simulink model "LLC_Controller"  (R2022b)
settings: Solver=FixedStepDiscrete  StartTime=0.0  StopTime=Inf  FixedStep=(20e-6)  RelTol=1e-3  EnableMultiTasking=on
undefined symbols (not defined in the file): GPTRIP1SEL, GPTRIP2SEL, SCI_A_Transmit, SCI_A_Transmit_Current_Suffix, SCI_A_Transmit_Duty_Suffix, SCI_A_Transmit_Freq_Suffix, SCI_A_Transmit_NewVRegPoint_Suffix, SCI_A_Transmit_OCPFlag_Suffix, SCI_A_Transmit_OVPFlag_Suffix, SCI_A_Transmit_PFC_Suffix, SCI_A_Transmit_SS_Suffix, SCI_A_Transmit_TBPHS_Suffix, SCI_A_Transmit_VADC_Suffix, SCI_A_Transmit_VAvg_Suffix, SCI_A_Transmit_VBAT_Suffix, SCI_A_Transmit_VBATRef_Suffix, SCI_A_Transmit_Vo_Suffix, TZ1, TZ2
libraries: c280xlib x16, c28003xlib x13, c2802xlib x8, simulink x7, c2837xDlib x3, c2000lib x1
(part 1 of 2)
settings Model: ExtModeTrigDuration=8  Creator=sgcesuser1  LastModifiedBy=sgcesuser1
settings SolverCC: AutoInsertRateTranBlk=on
settings DataIOCC: LimitDataPoints=on  SaveOutput=off  SaveTime=off  ReturnWorkspaceOutputs=off
settings OptimizationCC: DefaultUnderspecifiedDataType=single  EnhancedBackFolding=on  PassReuseOutputArgsAs=Individual arguments  MaxStackSize=1024  OptimizeBlockOrder=speed  DifferentSizesBufferReuse=on  OptimizationCustomize=off  DenormalBehavior=FlushToZero  EfficientTunableParamExpr=on
settings DebuggingCC: SolverPrmCheckMsg=warning  MultiTaskDSMMsg=none  MultiTaskCondExecSysMsg=none  ParameterTunabilityLossMsg=error  UnconnectedInputMsg=warning  UnconnectedOutputMsg=warning  UnconnectedLineMsg=warning  StateNameClashWarn=warning  SFUnexpectedBacktrackingDiag=warning  SFNoUnconditionalDefaultTransitionDiag=warning
settings HardwareCC: ProdBitPerChar=16  ProdBitPerInt=16  ProdBitPerPointer=32  ProdBitPerSizeT=32  ProdBitPerPtrDiffT=32  ProdLargestAtomicInteger=Integer  ProdLargestAtomicFloat=None  ProdWordSize=16  ProdLongLongMode=on  ProdHWDeviceType=Texas Instruments->C2000
settings ModelReferenceCC: EnableRefExpFcnMdlSchedulingChecks=on  PropagateSignalLabelsOutOfModel=off
settings SFSimCC: MATLABDynamicMemAlloc=off
settings RTWCC: Description=Embedded Coder  SystemTargetFile=ert.tlc  HardwareBoard=TI F28003x  TLCOptions=-aInlineSetEventsForThisBaseRateFcn=TLC_FALSE -aSuppressMultiTaskScheduler=TLC_FALSE -aRateBasedStepFcn=1  TemplateMakefile=ert_default_tmf  GenerateReport=on  Toolchain=Texas Instruments Code Composer Studio (C2000)  LaunchReport=on
settings CodeAppCC: IgnoreCustomStorageClasses=off  StateflowObjectComments=on
settings ERTTargetCC: CodeReplacementLibrary=TI C28x  ExtModeTransport=4  ExtModeStaticAlloc=on  ExtModeMexFile=ext_xcp  ExtModeIntrfLevel=Level2 - Open  ConvertIfToSwitch=off  SuppressUnreachableDefaultCases=off

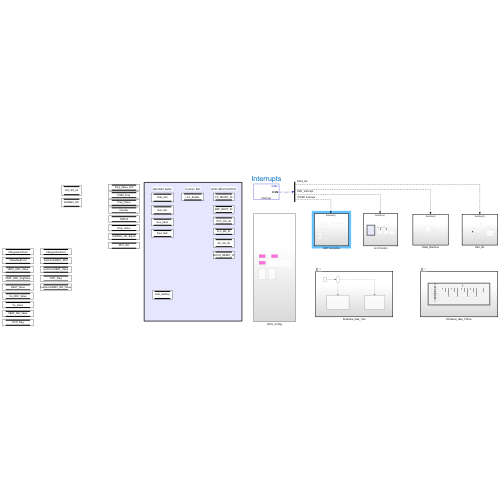
[thumbnail: Simulink's stored preview of the top-level diagram]
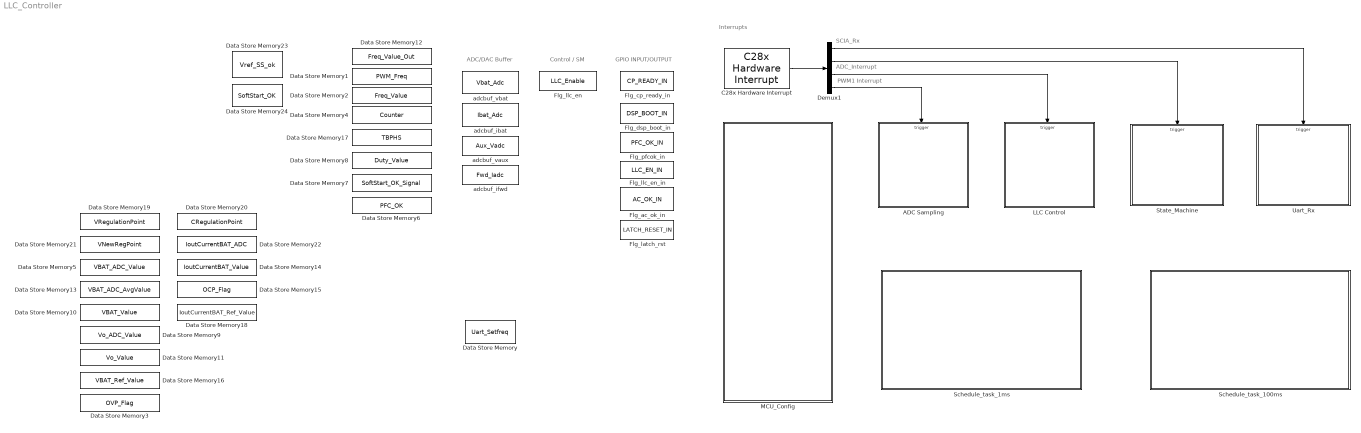
== system LLC_Controller ==
  note: ADC_Interrupt
  note: PWM1 Interrupt
  note: Interrupts
  note: GPIO INPUT/OUTPUT
  note: ADC/DAC Buffer
  note: Control / SM
  note: SCIA_Rx
  ADC Sampling : Subsystem  TreatAsAtomicUnit=on
  C28x Hardware Interrupt : c2000lib/Scheduling/C28x Hardware Interrupt  irqnumbers=[9 3 1 3]  pienumbers=[1 8 3 1]  irqpriorities=[33 32 30 31]  irqpreempts=[1 1 0 0]  showinput=off  dspchiptype=C280X
  Data Store Memory : DataStoreMemory  DataStoreName=Uart_Setfreq  WriteAfterWriteMsg=warning  InitialValue=100  ShowAdditionalParam=off  OutDataTypeStr=single
  Data Store Memory1 : DataStoreMemory  DataStoreName=PWM_Freq  WriteAfterWriteMsg=warning  ShowAdditionalParam=off  OutDataTypeStr=double
  Data Store Memory10 : DataStoreMemory  DataStoreName=VBAT_Value  WriteAfterWriteMsg=warning  ShowAdditionalParam=off  OutDataTypeStr=double
  Data Store Memory11 : DataStoreMemory  DataStoreName=Vo_Value  WriteAfterWriteMsg=warning  InitialValue=153  ShowAdditionalParam=off
  Data Store Memory12 : DataStoreMemory  DataStoreName=Freq_Value_Out  WriteAfterWriteMsg=warning  InitialValue=153  ShowAdditionalParam=off  OutDataTypeStr=double
  Data Store Memory13 : DataStoreMemory  DataStoreName=VBAT_ADC_AvgValue  WriteAfterWriteMsg=warning  ShowAdditionalParam=off
  Data Store Memory14 : DataStoreMemory  DataStoreName=IoutCurrentBAT_Value  WriteAfterWriteMsg=warning  ShowAdditionalParam=off  OutDataTypeStr=double
  Data Store Memory15 : DataStoreMemory  DataStoreName=OCP_Flag  WriteAfterWriteMsg=warning  InitialValue=1  ShowAdditionalParam=off
  Data Store Memory16 : DataStoreMemory  DataStoreName=VBAT_Ref_Value  WriteAfterWriteMsg=warning  ShowAdditionalParam=off  OutDataTypeStr=double
  Data Store Memory17 : DataStoreMemory  DataStoreName=TBPHS  WriteAfterWriteMsg=warning  ShowAdditionalParam=off  OutDataTypeStr=double
  Data Store Memory18 : DataStoreMemory  DataStoreName=IoutCurrentBAT_Ref_Value  WriteAfterWriteMsg=warning  ShowAdditionalParam=off  OutDataTypeStr=double
  Data Store Memory19 : DataStoreMemory  DataStoreName=VRegulationPoint  WriteAfterWriteMsg=warning  ShowAdditionalParam=off  OutDataTypeStr=double
  Data Store Memory2 : DataStoreMemory  DataStoreName=Freq_Value  WriteAfterWriteMsg=warning  InitialValue=153  ShowAdditionalParam=off  OutDataTypeStr=double
  Data Store Memory20 : DataStoreMemory  DataStoreName=CRegulationPoint  WriteAfterWriteMsg=warning  ShowAdditionalParam=off  OutDataTypeStr=double
  Data Store Memory21 : DataStoreMemory  DataStoreName=VNewRegPoint  WriteAfterWriteMsg=warning  ShowAdditionalParam=off  OutDataTypeStr=double
  Data Store Memory22 : DataStoreMemory  DataStoreName=IoutCurrentBAT_ADC  WriteAfterWriteMsg=warning  ShowAdditionalParam=off  OutDataTypeStr=double
  Data Store Memory23 : DataStoreMemory  DataStoreName=Vref_SS_ok  WriteAfterWriteMsg=warning  ShowAdditionalParam=off
  Data Store Memory24 : DataStoreMemory  DataStoreName=SoftStart_OK  WriteAfterWriteMsg=warning  ShowAdditionalParam=off
  Data Store Memory3 : DataStoreMemory  DataStoreName=OVP_Flag  WriteAfterWriteMsg=warning  InitialValue=1  ShowAdditionalParam=off
  Data Store Memory4 : DataStoreMemory  DataStoreName=Counter  WriteAfterWriteMsg=warning  InitialValue=153  ShowAdditionalParam=off
  Data Store Memory5 : DataStoreMemory  DataStoreName=VBAT_ADC_Value  WriteAfterWriteMsg=warning  InitialValue=153  ShowAdditionalParam=off  OutDataTypeStr=double
  Data Store Memory6 : DataStoreMemory  DataStoreName=PFC_OK  WriteAfterWriteMsg=warning  ShowAdditionalParam=off
  Data Store Memory7 : DataStoreMemory  DataStoreName=SoftStart_OK_Signal  WriteAfterWriteMsg=warning  ShowAdditionalParam=off
  Data Store Memory8 : DataStoreMemory  DataStoreName=Duty_Value  WriteAfterWriteMsg=warning  InitialValue=1  ShowAdditionalParam=off  OutDataTypeStr=double
  Data Store Memory9 : DataStoreMemory  DataStoreName=Vo_ADC_Value  WriteAfterWriteMsg=warning  InitialValue=153  ShowAdditionalParam=off
  Demux1 : Demux
  Flg_ac_ok_in : DataStoreMemory  DataStoreName=AC_OK_IN  WriteAfterWriteMsg=warning  ShowAdditionalParam=off
  Flg_cp_ready_in : DataStoreMemory  DataStoreName=CP_READY_IN  WriteAfterWriteMsg=warning  ShowAdditionalParam=off
  Flg_dsp_boot_in : DataStoreMemory  DataStoreName=DSP_BOOT_IN  WriteAfterWriteMsg=warning  ShowAdditionalParam=off
  Flg_latch_rst : DataStoreMemory  DataStoreName=LATCH_RESET_IN  WriteAfterWriteMsg=warning  ShowAdditionalParam=off
  Flg_llc_en : DataStoreMemory  DataStoreName=LLC_Enable  WriteAfterWriteMsg=warning  ShowAdditionalParam=off  OutDataTypeStr=boolean
  Flg_llc_en_in : DataStoreMemory  DataStoreName=LLC_EN_IN  WriteAfterWriteMsg=warning  ShowAdditionalParam=off
  Flg_pfcok_in : DataStoreMemory  DataStoreName=PFC_OK_IN  WriteAfterWriteMsg=warning  ShowAdditionalParam=off
  LLC Control : Subsystem  TreatAsAtomicUnit=on
  MCU_Config : Subsystem
  Schedule_task_100ms : Subsystem  TreatAsAtomicUnit=on  ScheduleAs=Periodic partition  PartitionName=Schedule_task_100ms  SystemSampleTime=1
  Schedule_task_1ms : Subsystem  TreatAsAtomicUnit=on  ScheduleAs=Periodic partition  PartitionName=Schedule_task_1ms  SystemSampleTime=0.001
  State_Machine : Subsystem  TreatAsAtomicUnit=on
  Uart_Rx : Subsystem  TreatAsAtomicUnit=on
  adcbuf_ibat : DataStoreMemory  DataStoreName=Ibat_Adc  WriteAfterWriteMsg=warning  ShowAdditionalParam=off  OutDataTypeStr=uint16
  adcbuf_ifwd : DataStoreMemory  DataStoreName=Fwd_Iadc  WriteAfterWriteMsg=warning  ShowAdditionalParam=off  OutDataTypeStr=uint16
  adcbuf_vaux : DataStoreMemory  DataStoreName=Aux_Vadc  WriteAfterWriteMsg=warning  ShowAdditionalParam=off  OutDataTypeStr=uint16
  adcbuf_vbat : DataStoreMemory  DataStoreName=Vbat_Adc  WriteAfterWriteMsg=warning  ShowAdditionalParam=off  OutDataTypeStr=uint16
  wires:
  C28x Hardware Interrupt/1 -> Demux1/1
  Demux1/3 -> LLC Control/Trigger
  Demux1/4 -> ADC Sampling/Trigger
  Demux1/2 -> State_Machine/Trigger
  Demux1/1 -> Uart_Rx/Trigger

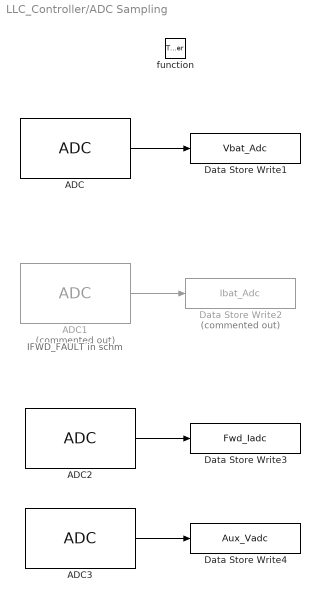
== system LLC_Controller/ADC Sampling ==
  note: IFWD_FAULT in schm
  function : TriggerPort  TriggerType=function-call  VariantControl=(inherit)
  ADC : c2802xlib/ADC  blkParamProc=C2000_Type5  ADCModule=C  samplingMode=Single sample mode  ADCResolution=12-bit (Single-ended input)  useSOC1=SOC0  useSOC2=SOC0_SOC1  SOCAcquisitionWindow=8  SOCTriggerSource=Software  SOCInterruptTrigger=No ADCINT  Ts=-1  dType=uint16  postInterrupt=on  interruptSel=ADCINT1  ADCINTContinuous=on  endma=off  chdma=1  conv1=ADCINA0  conv2=ADCINA0 and ADCINB0  conv1_Type4=ADCIN5  conv2_Type4=ADCIN0 and ADCIN1
  ADC1 : c2802xlib/ADC  Commented=on  blkParamProc=C2000_Type5  ADCModule=A  samplingMode=Single sample mode  ADCResolution=12-bit (Single-ended input)  useSOC1=SOC2  useSOC2=SOC0_SOC1  SOCAcquisitionWindow=8  SOCTriggerSource=Software  SOCInterruptTrigger=No ADCINT  Ts=-1  dType=uint16  postInterrupt=off  interruptSel=ADCINT1  ADCINTContinuous=off  endma=off  chdma=1  conv1=ADCINA0  conv2=ADCINA0 and ADCINB0  conv1_Type4=ADCIN9  conv2_Type4=ADCIN0 and ADCIN1
  ADC2 : c2802xlib/ADC  blkParamProc=C2000_Type5  ADCModule=B  samplingMode=Single sample mode  ADCResolution=12-bit (Single-ended input)  useSOC1=SOC0  useSOC2=SOC0_SOC1  SOCAcquisitionWindow=8  SOCTriggerSource=Software  SOCInterruptTrigger=No ADCINT  Ts=-1  dType=uint16  postInterrupt=off  interruptSel=ADCINT1  ADCINTContinuous=off  endma=off  chdma=1  conv1=ADCINA0  conv2=ADCINA0 and ADCINB0  conv1_Type4=ADCIN11  conv2_Type4=ADCIN0 and ADCIN1
  ADC3 : c2802xlib/ADC  blkParamProc=C2000_Type5  ADCModule=C  samplingMode=Single sample mode  ADCResolution=12-bit (Single-ended input)  useSOC1=SOC2  useSOC2=SOC0_SOC1  SOCAcquisitionWindow=8  SOCTriggerSource=Software  SOCInterruptTrigger=No ADCINT  Ts=-1  dType=uint16  postInterrupt=off  interruptSel=ADCINT1  ADCINTContinuous=off  endma=off  chdma=1  conv1=ADCINA0  conv2=ADCINA0 and ADCINB0  conv1_Type4=ADCIN1  conv2_Type4=ADCIN0 and ADCIN1
  Data Store Write1 : DataStoreWrite  DataStoreName=Vbat_Adc  IndexOptions=Index vector (dialog)  Indices=1  OutputSizes=1
  Data Store Write2 : DataStoreWrite  Commented=on  DataStoreName=Ibat_Adc  IndexOptions=Index vector (dialog)  Indices=1  OutputSizes=1
  Data Store Write3 : DataStoreWrite  DataStoreName=Fwd_Iadc  IndexOptions=Index vector (dialog)  Indices=1  OutputSizes=1
  Data Store Write4 : DataStoreWrite  DataStoreName=Aux_Vadc  IndexOptions=Index vector (dialog)  Indices=1  OutputSizes=1
  wires:
  ADC/1 -> Data Store Write1/1
  ADC1/1 -> Data Store Write2/1
  ADC2/1 -> Data Store Write3/1
  ADC3/1 -> Data Store Write4/1

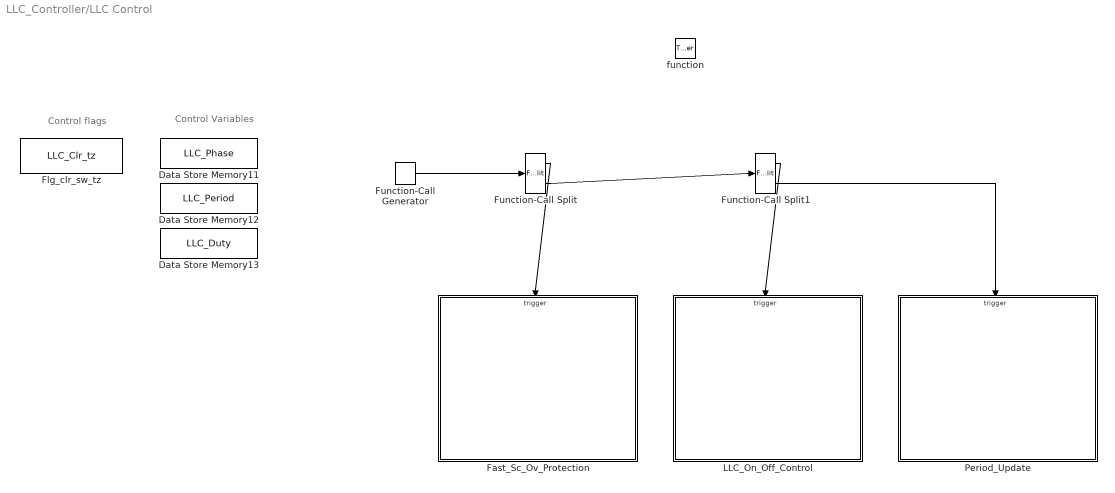
== system LLC_Controller/LLC Control ==
  note: Control flags
  note: Control Variables
  function : TriggerPort  TriggerType=function-call  VariantControl=(inherit)
  Data Store Memory11 : DataStoreMemory  DataStoreName=LLC_Phase  WriteAfterWriteMsg=warning  InitialValue=300  ShowAdditionalParam=off  OutDataTypeStr=single
  Data Store Memory12 : DataStoreMemory  DataStoreName=LLC_Period  WriteAfterWriteMsg=warning  InitialValue=(120e6)/(300e3)  ShowAdditionalParam=off  OutDataTypeStr=single
  Data Store Memory13 : DataStoreMemory  DataStoreName=LLC_Duty  WriteAfterWriteMsg=warning  InitialValue=(100/50)  ShowAdditionalParam=off  OutDataTypeStr=single
  Fast_Sc_Ov_Protection : Subsystem  TreatAsAtomicUnit=on
  Flg_clr_sw_tz : DataStoreMemory  DataStoreName=LLC_Clr_tz  WriteAfterWriteMsg=warning  ShowAdditionalParam=off  OutDataTypeStr=boolean
  Function-Call Generator : simulink/Ports & Subsystems/Function-Call Generator  sample_time=-1  numberOfIterations=1  DisallowWideOutput=off
  Function-Call Split : FunctionCallSplit  NumOutputPorts=2
  Function-Call Split1 : FunctionCallSplit  NumOutputPorts=2
  LLC_On_Off_Control : Subsystem  TreatAsAtomicUnit=on
  Period_Update : Subsystem  TreatAsAtomicUnit=on
  wires:
  Function-Call Generator/1 -> Function-Call Split/1
  Function-Call Split/1 -> Fast_Sc_Ov_Protection/Trigger
  Function-Call Split1/1 -> LLC_On_Off_Control/Trigger
  Function-Call Split/2 -> Function-Call Split1/1
  Function-Call Split1/2 -> Period_Update/Trigger

== system LLC_Controller/MCU_Config ==
  note: EALLOW;
      | EPwm5Regs.EPWMSYNCOUTEN.all = 0x02;  //PWM5 SYNCOUT signal at TBCTR = 0
      | EPwm7Regs.EPWMSYNCINSEL.all = 0x05;    //PWM7 SYNCIN to PWM5
      | EPwm5Regs.TZSEL.bit.OSHT1 = 1;
      | EPwm7Regs.TZSEL.bit.OSHT1 = 1;
      | EPwm5Regs.TZFRC.bit.OST = 1;
      | EPwm7Regs.TZFRC.bit.OST = 1;
      | EDIS;
  ADC_TriggerSource : c2802xlib/ePWM  PwmType=C2000_Type4_F28002x  useModule=ePWM1  ePWMxLINKTBPRD=Not Linked  periodUnits=Seconds  timerSource=Specify via dialog  timerPeriod_clk=(120e6/50e3)  timerPeriod_sec=50e-6  tbshadow=Counter equals to zero  countingMode=Up  phaseActiveEnable=Disable  phaseDirection=Count down after sync  phaseActive=0  synchronizationEnable=off  dcaevt1Sync=off  dcbevt1Sync=off  synchronizationOption=Counter equals to zero (CTR=Zero)  dcbevt1SyncOut=off  dcaevt1SyncOut=off  cmpdSyncOut=off  cmpcSyncOut=off  cmpbSyncOut=off  zeroSyncOut=on  swfSyncOut=off  perSynchronizationOption=Counter equals to period (CTR=PRD)  clockPrescale=1  HSclockPrescale=1  enswap=off  ePWMxAStatus=off  ePWMxAactionLogic1=Set  ePWMxAactionLogic2=Do nothing  ePWMxAactionLogic3=Clear  ePWMxAactionLogic4=Do nothing  ePWMxAactionLogic5=Do nothing  ePWMxAactionLogic6=Do nothing  ePWMxACSFenable=off  ePWMxACSFvalue=Forcing disable  ePWMxASFreload=Zero  ePWMxBStatus=off  ePWMxBactionLogic1=Clear  ePWMxBactionLogic2=Do nothing  ePWMxBactionLogic3=Set  ePWMxBactionLogic4=Do nothing  ePWMxBactionLogic5=Do nothing  ePWMxBactionLogic6=Set  ePWMxBCSFenable=off  ePWMxBCSFvalue=Forcing disable  ePWMxBSFreload=Zero  ePWNxBOutWay=off  ePWMxLINKCMPA=Not Linked  CMPAUnits=Clock cycles  CMPASource=Specify via dialog  CMPAValue_per=50  CMPAValue_clk=50  enCMPAshadow=Counter equals to zero (CTR=Zero)  ePWMxLINKCMPB=Not Linked  CMPBUnits=Clock cycles  CMPBSource=Specify via dialog  CMPBValue_per=50  CMPBValue_clk=1000  enCMPBshadow=Counter equals to zero (CTR=Zero)  ePWMxLINKCMPC=Not Linked  CMPCUnits=Clock cycles  CMPCSource=Specify via dialog  CMPCValue_per=50  CMPCValue_clk=32000  enCMPCshadow=Counter equals to zero (CTR=Zero)  ePWMxLINKCMPD=Not Linked  CMPDUnits=Percentages  CMPDSource=Specify via dialog  CMPDValue_per=50  CMPDValue_clk=32000  enCMPDshadow=Counter equals to zero (CTR=Zero)  enableDBePWMxA=off  enableDBePWMxB=off  enhalfcycle=off  DBpolarity=Active high complementary (AHC)  DBedgeDelay=Positive  DBSource_ePWMxA=ePWMxA  DBSource_ePWMxB=ePWMxA  DBPeriodUnits=Seconds  DBperiodSource=Specify via dialog  REDperiod=0  FEDperiod=0  REDperiod_sec=250e-9  FEDperiod_sec=250e-9  LoadModeDBRED=Counter equals to zero (CTR=ZERO)  LoadModeDBFED=Counter equals to zero (CTR=ZERO)  adcstartModuleA=off  adcrequestEventA=First event  adcstartEventA=Counter equals to zero (CTR=Zero)  adcstartEventA_type2=Counter equals to zero (CTR=Zero)  adcstartModuleB=off  adcrequestEventB=First event  adcstartEventB=Counter equals to zero (CTR=Zero)  adcstartEventB_type2=Counter equals to zero (CTR=Zero)  intEn=on  intPrd=First event  intSel=Counter equals to zero (CTR=Zero)  intSel_type2=Counter equals to zero (CTR=Zero)  hrpe=off  enHRPWM=off  HRPWM_LoadMode=Counter equals to zero (CTR=ZERO)  HRPWM_CTLMode=Duty or Period control mode  HRPWM_EDGMode=Both edge  hrpeb=off  enHRPWMB=off  HRPWM_LoadModeB=Counter equals to zero (CTR=ZERO)  HRPWM_CTLModeB=Duty or Period control mode  HRPWM_EDGModeB=Both edge  enHRDBRED=off  enHRDBFED=off  enSFO=on  enautoconv=on  chopperEnable=off  chopperFrequency=1  chopperFirstwidth=1  chopperDuty=12.5%  tripZonesource=Specify via dialog  tzselOSHT1=off  tzselOSHT2=off  tzselOSHT3=off  tzselOSHDCAEV1=off  tzselOSHDCBEV1=off  tzselCBC1=off  tzselCBC2=off  tzselCBC3=off  tzselCBCDCAEV2=off  tzselCBCDCBEV2=off  tzselOSHT4=off  tzselOSHT5=off  tzselOSHT6=off  tzselCBC4=off  tzselCBC5=off  tzselCBC6=off  enTzOstIntr=off  enTzCbcIntr=off  enTzDCAEVT1Intr=off  enTzDCAEVT2Intr=off  enTzDCBEVT1Intr=off  enTzDCBEVT2Intr=off  ePWMxAforced=No action  ePWMxBforced=No action  DCAEVT1forced=No action  DCBEVT1forced=No action  DCAEVT2forced=No action  DCBEVT2forced=No action  dcah=Trip Zone 1 input (TZ1)  dcal=Trip Zone 1 input (TZ1)  dcbh=Trip Zone 1 input (TZ1)  dcbl=Trip Zone 1 input (TZ1)  dcah_type2=GPTRIP1SEL/(TZ1)  dcal_type2=GPTRIP2SEL/(TZ2)  dcbh_type2=GPTRIP1SEL/(TZ1)  dcbl_type2=GPTRIP2SEL/(TZ2)  gendcaevt1=Event disabled  gendcaevt2=Event disabled  gendcbevt1=Event disabled  gendcbevt2=Event disabled  dcaevt1src=DCAEVT1 with sync  dcaevt2src=DCAEVT2 with sync  dcbevt1src=DCBEVT1 with sync  dcbevt2src=DCBEVT2 with sync  pulsesel=Counter equals to zero (CTR=Zero)  blankinv=off  blankoffset=0  blankwidth=0  evsrcsel=Filtered version of DCAEVT1 (DCAEVT1FILT)  encape=off
  CMPSS/ANALOG Initialize : Subsystem  mask(System Initialize){ShowInLibBrowser=0}
      mask prompts: ShowInLibBrowser "Simulink:masks:CustCodeMaskParam1_MP"
      settings: CopyFcn=cccopyfcn(gcb)  OpenFcn=ccopenfcn('System Initialize Function')
      mask Help: eval('feval(''rtwprivate'',''rtwhelpview'',''rtw_sys_initialize_block'')');
      mask Display: disp('System\nInitialize');
  PWM Initialize : Subsystem  mask(System Initialize){ShowInLibBrowser=0}
      mask prompts: ShowInLibBrowser "Simulink:masks:CustCodeMaskParam1_MP"
      settings: CopyFcn=cccopyfcn(gcb)  OpenFcn=ccopenfcn('System Initialize Function')
      mask Help: eval('feval(''rtwprivate'',''rtwhelpview'',''rtw_sys_initialize_block'')');
      mask Display: disp('System\nInitialize');
  StateMachine_Int : c2802xlib/ePWM  PwmType=C2000_Type4_F28002x  useModule=ePWM8  ePWMxLINKTBPRD=Not Linked  periodUnits=Seconds  timerSource=Specify via dialog  timerPeriod_clk=(120e6/50e3)  timerPeriod_sec=200e-6  tbshadow=Counter equals to zero  countingMode=Up  phaseActiveEnable=Disable  phaseDirection=Count down after sync  phaseActive=0  synchronizationEnable=off  dcaevt1Sync=off  dcbevt1Sync=off  synchronizationOption=Counter equals to zero (CTR=Zero)  dcbevt1SyncOut=off  dcaevt1SyncOut=off  cmpdSyncOut=off  cmpcSyncOut=off  cmpbSyncOut=off  zeroSyncOut=on  swfSyncOut=off  perSynchronizationOption=Counter equals to period (CTR=PRD)  clockPrescale=1  HSclockPrescale=1  enswap=off  ePWMxAStatus=off  ePWMxAactionLogic1=Set  ePWMxAactionLogic2=Do nothing  ePWMxAactionLogic3=Clear  ePWMxAactionLogic4=Do nothing  ePWMxAactionLogic5=Do nothing  ePWMxAactionLogic6=Do nothing  ePWMxACSFenable=off  ePWMxACSFvalue=Forcing disable  ePWMxASFreload=Zero  ePWMxBStatus=off  ePWMxBactionLogic1=Clear  ePWMxBactionLogic2=Do nothing  ePWMxBactionLogic3=Set  ePWMxBactionLogic4=Do nothing  ePWMxBactionLogic5=Do nothing  ePWMxBactionLogic6=Set  ePWMxBCSFenable=off  ePWMxBCSFvalue=Forcing disable  ePWMxBSFreload=Zero  ePWNxBOutWay=off  ePWMxLINKCMPA=Not Linked  CMPAUnits=Clock cycles  CMPASource=Specify via dialog  CMPAValue_per=50  CMPAValue_clk=50  enCMPAshadow=Counter equals to zero (CTR=Zero)  ePWMxLINKCMPB=Not Linked  CMPBUnits=Clock cycles  CMPBSource=Specify via dialog  CMPBValue_per=50  CMPBValue_clk=1000  enCMPBshadow=Counter equals to zero (CTR=Zero)  ePWMxLINKCMPC=Not Linked  CMPCUnits=Clock cycles  CMPCSource=Specify via dialog  CMPCValue_per=50  CMPCValue_clk=32000  enCMPCshadow=Counter equals to zero (CTR=Zero)  ePWMxLINKCMPD=Not Linked  CMPDUnits=Percentages  CMPDSource=Specify via dialog  CMPDValue_per=50  CMPDValue_clk=32000  enCMPDshadow=Counter equals to zero (CTR=Zero)  enableDBePWMxA=off  enableDBePWMxB=off  enhalfcycle=off  DBpolarity=Active high complementary (AHC)  DBedgeDelay=Positive  DBSource_ePWMxA=ePWMxA  DBSource_ePWMxB=ePWMxA  DBPeriodUnits=Seconds  DBperiodSource=Specify via dialog  REDperiod=0  FEDperiod=0  REDperiod_sec=250e-9  FEDperiod_sec=250e-9  LoadModeDBRED=Counter equals to zero (CTR=ZERO)  LoadModeDBFED=Counter equals to zero (CTR=ZERO)  adcstartModuleA=off  adcrequestEventA=First event  adcstartEventA=Counter equals to zero (CTR=Zero)  adcstartEventA_type2=Counter equals to zero (CTR=Zero)  adcstartModuleB=off  adcrequestEventB=First event  adcstartEventB=Counter equals to zero (CTR=Zero)  adcstartEventB_type2=Counter equals to zero (CTR=Zero)  intEn=on  intPrd=First event  intSel=Counter equals to zero (CTR=Zero)  intSel_type2=Counter equals to zero (CTR=Zero)  hrpe=off  enHRPWM=off  HRPWM_LoadMode=Counter equals to zero (CTR=ZERO)  HRPWM_CTLMode=Duty or Period control mode  HRPWM_EDGMode=Both edge  hrpeb=off  enHRPWMB=off  HRPWM_LoadModeB=Counter equals to zero (CTR=ZERO)  HRPWM_CTLModeB=Duty or Period control mode  HRPWM_EDGModeB=Both edge  enHRDBRED=off  enHRDBFED=off  enSFO=on  enautoconv=on  chopperEnable=off  chopperFrequency=1  chopperFirstwidth=1  chopperDuty=12.5%  tripZonesource=Specify via dialog  tzselOSHT1=off  tzselOSHT2=off  tzselOSHT3=off  tzselOSHDCAEV1=off  tzselOSHDCBEV1=off  tzselCBC1=off  tzselCBC2=off  tzselCBC3=off  tzselCBCDCAEV2=off  tzselCBCDCBEV2=off  tzselOSHT4=off  tzselOSHT5=off  tzselOSHT6=off  tzselCBC4=off  tzselCBC5=off  tzselCBC6=off  enTzOstIntr=off  enTzCbcIntr=off  enTzDCAEVT1Intr=off  enTzDCAEVT2Intr=off  enTzDCBEVT1Intr=off  enTzDCBEVT2Intr=off  ePWMxAforced=No action  ePWMxBforced=No action  DCAEVT1forced=No action  DCBEVT1forced=No action  DCAEVT2forced=No action  DCBEVT2forced=No action  dcah=Trip Zone 1 input (TZ1)  dcal=Trip Zone 1 input (TZ1)  dcbh=Trip Zone 1 input (TZ1)  dcbl=Trip Zone 1 input (TZ1)  dcah_type2=GPTRIP1SEL/(TZ1)  dcal_type2=GPTRIP2SEL/(TZ2)  dcbh_type2=GPTRIP1SEL/(TZ1)  dcbl_type2=GPTRIP2SEL/(TZ2)  gendcaevt1=Event disabled  gendcaevt2=Event disabled  gendcbevt1=Event disabled  gendcbevt2=Event disabled  dcaevt1src=DCAEVT1 with sync  dcaevt2src=DCAEVT2 with sync  dcbevt1src=DCBEVT1 with sync  dcbevt2src=DCBEVT2 with sync  pulsesel=Counter equals to zero (CTR=Zero)  blankinv=off  blankoffset=0  blankwidth=0  evsrcsel=Filtered version of DCAEVT1 (DCAEVT1FILT)  encape=off

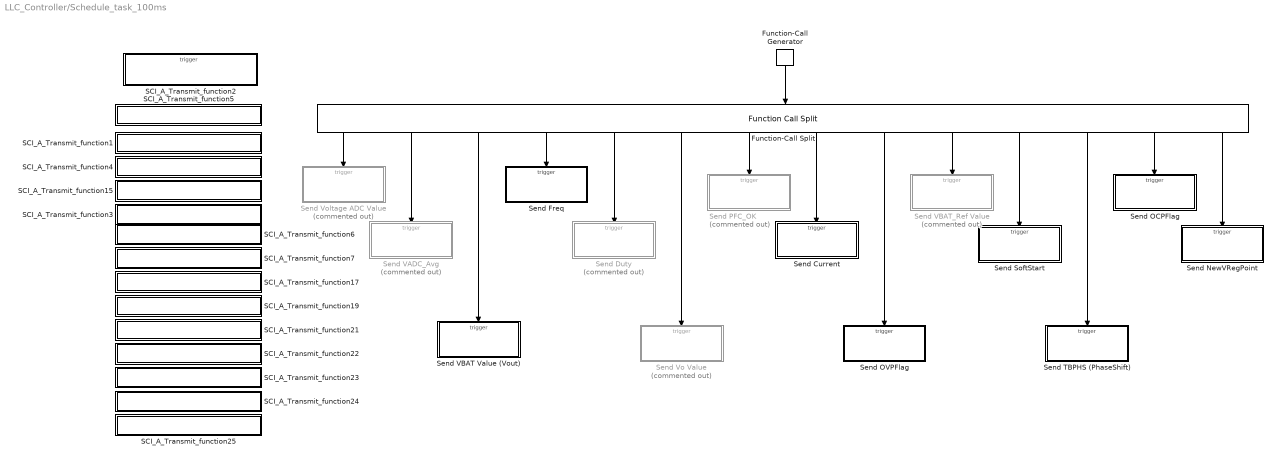
== system LLC_Controller/Schedule_task_100ms ==
  Function-Call Generator : simulink/Ports & Subsystems/Function-Call Generator  sample_time=-1  numberOfIterations=1  DisallowWideOutput=off
  Function-Call Split : FunctionCallSplit  IconShape=distinctive  NumOutputPorts=14  OutputPortLayout=default
  SCI_A_Transmit_function1 : Subsystem  TreatAsAtomicUnit=on
  SCI_A_Transmit_function15 : Subsystem  TreatAsAtomicUnit=on
  SCI_A_Transmit_function17 : Subsystem  TreatAsAtomicUnit=on
  SCI_A_Transmit_function19 : Subsystem  TreatAsAtomicUnit=on
  SCI_A_Transmit_function2 : Subsystem  TreatAsAtomicUnit=on
  SCI_A_Transmit_function21 : Subsystem  TreatAsAtomicUnit=on
  SCI_A_Transmit_function22 : Subsystem  TreatAsAtomicUnit=on
  SCI_A_Transmit_function23 : Subsystem  TreatAsAtomicUnit=on
  SCI_A_Transmit_function24 : Subsystem  TreatAsAtomicUnit=on
  SCI_A_Transmit_function25 : Subsystem  TreatAsAtomicUnit=on
  SCI_A_Transmit_function3 : Subsystem  TreatAsAtomicUnit=on
  SCI_A_Transmit_function4 : Subsystem  TreatAsAtomicUnit=on
  SCI_A_Transmit_function5 : Subsystem  TreatAsAtomicUnit=on
  SCI_A_Transmit_function6 : Subsystem  TreatAsAtomicUnit=on
  SCI_A_Transmit_function7 : Subsystem  TreatAsAtomicUnit=on
  Send Current : Subsystem  TreatAsAtomicUnit=on
  Send Duty : Subsystem  Commented=on  TreatAsAtomicUnit=on
  Send Freq : Subsystem  TreatAsAtomicUnit=on
  Send NewVRegPoint : Subsystem  TreatAsAtomicUnit=on
  Send OCPFlag : Subsystem  TreatAsAtomicUnit=on
  Send OVPFlag : Subsystem  TreatAsAtomicUnit=on
  Send PFC_OK : Subsystem  Commented=on  TreatAsAtomicUnit=on
  Send SoftStart : Subsystem  TreatAsAtomicUnit=on
  Send TBPHS (PhaseShift) : Subsystem  TreatAsAtomicUnit=on
  Send VADC_Avg : Subsystem  Commented=on  TreatAsAtomicUnit=on
  Send VBAT Value (Vout) : Subsystem  TreatAsAtomicUnit=on
  Send VBAT_Ref Value : Subsystem  Commented=on  TreatAsAtomicUnit=on
  Send Vo Value : Subsystem  Commented=on  TreatAsAtomicUnit=on
  Send Voltage ADC Value : Subsystem  Commented=on  TreatAsAtomicUnit=on
  wires:
  Function-Call Split/13 -> Send OCPFlag/Trigger
  Function-Call Split/12 -> Send TBPHS (PhaseShift)/Trigger
  Function-Call Split/5 -> Send Duty/Trigger
  Function-Call Split/14 -> Send NewVRegPoint/Trigger
  Function-Call Split/9 -> Send OVPFlag/Trigger
  Function-Call Split/4 -> Send Freq/Trigger
  Function-Call Split/3 -> Send VBAT Value (Vout)/Trigger
  Function-Call Split/6 -> Send Vo Value/Trigger
  Function-Call Split/11 -> Send SoftStart/Trigger
  Function-Call Split/8 -> Send Current/Trigger
  Function-Call Generator/1 -> Function-Call Split/1
  Function-Call Split/10 -> Send VBAT_Ref Value/Trigger
  Function-Call Split/2 -> Send VADC_Avg/Trigger
  Function-Call Split/7 -> Send PFC_OK/Trigger
  Function-Call Split/1 -> Send Voltage ADC Value/Trigger

== system LLC_Controller/Schedule_task_1ms ==
  Function-Call Generator : simulink/Ports & Subsystems/Function-Call Generator  sample_time=-1  numberOfIterations=1  DisallowWideOutput=off
  Function-Call Split : FunctionCallSplit  NumOutputPorts=2
  Function-Call Subsystem1 : Subsystem  TreatAsAtomicUnit=on
  Gpio_Update : Subsystem  TreatAsAtomicUnit=on
  wires:
  Function-Call Generator/1 -> Function-Call Split/1
  Function-Call Split/1 -> Gpio_Update/Trigger
  Function-Call Split/2 -> Function-Call Subsystem1/Trigger

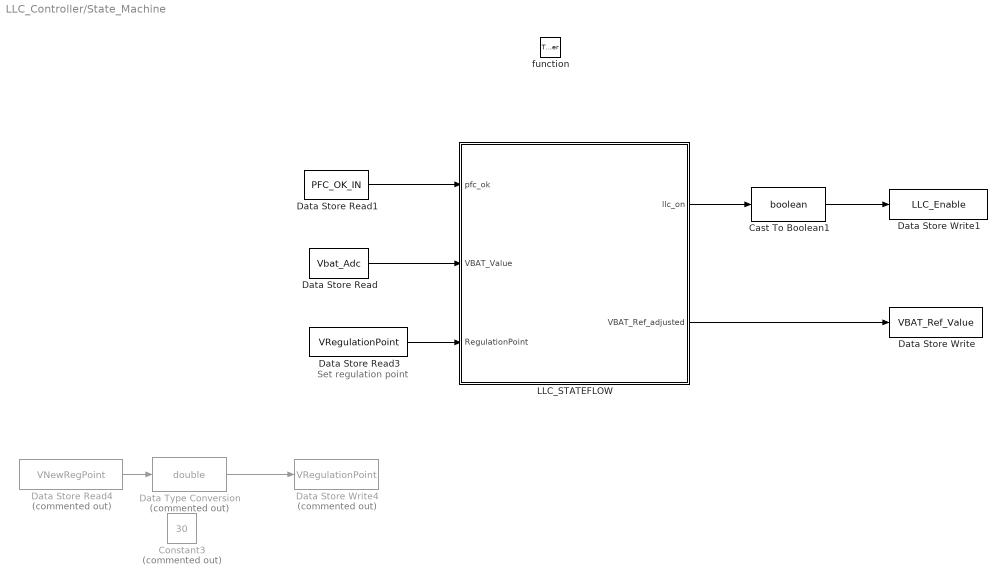
== system LLC_Controller/State_Machine ==
  note: Set regulation point
  function : TriggerPort  TriggerType=function-call  VariantControl=(inherit)
  Cast To Boolean1 : DataTypeConversion  OutDataTypeStr=boolean  SaturateOnIntegerOverflow=off  RndMeth=Floor
  Constant3 : Constant  Commented=on  Value=30  OutDataTypeStr=double  SampleTime=Inf
  Data Store Read : DataStoreRead  DataStoreName=Vbat_Adc  IndexOptions=Index vector (dialog)  Indices=1  OutputSizes=1
  Data Store Read1 : DataStoreRead  DataStoreName=PFC_OK_IN  IndexOptions=Index vector (dialog)  Indices=1  OutputSizes=1
  Data Store Read3 : DataStoreRead  DataStoreName=VRegulationPoint  IndexOptions=Index vector (dialog)  Indices=1  OutputSizes=1
  Data Store Read4 : DataStoreRead  Commented=on  DataStoreName=VNewRegPoint  IndexOptions=Index vector (dialog)  Indices=1  OutputSizes=1
  Data Store Write : DataStoreWrite  DataStoreName=VBAT_Ref_Value  IndexOptions=Index vector (dialog)  Indices=1  OutputSizes=1
  Data Store Write1 : DataStoreWrite  DataStoreName=LLC_Enable  IndexOptions=Index vector (dialog)  Indices=1  OutputSizes=1
  Data Store Write4 : DataStoreWrite  Commented=on  DataStoreName=VRegulationPoint  IndexOptions=Index vector (dialog)  Indices=1  OutputSizes=1
  Data Type Conversion : DataTypeConversion  Commented=on  OutDataTypeStr=double  SaturateOnIntegerOverflow=off  RndMeth=Floor
  LLC_STATEFLOW : Stateflow chart  TreatAsAtomicUnit=on
  wires:
  LLC_STATEFLOW/1(llc_on) -> Cast To Boolean1/1
  Data Store Read1/1 -> LLC_STATEFLOW/1(pfc_ok)
  Cast To Boolean1/1 -> Data Store Write1/1
  Data Store Read/1 -> LLC_STATEFLOW/2(VBAT_Value)
  Data Type Conversion/1 -> Data Store Write4/1
  Data Store Read4/1 -> Data Type Conversion/1
  Data Store Read3/1 -> LLC_STATEFLOW/3(RegulationPoint)
  LLC_STATEFLOW/2(VBAT_Ref_adjusted) -> Data Store Write/1

== system LLC_Controller/Uart_Rx ==
  note: Frequency Range Limited to 001K to 999K due to comparing 3 Digit
  function : TriggerPort  TriggerType=function-call  VariantControl=(inherit)
  Function-Call Generator : simulink/Ports & Subsystems/Function-Call Generator  sample_time=-1  numberOfIterations=1  DisallowWideOutput=off
  Function-Call Subsystem : Subsystem  TreatAsAtomicUnit=on
  Simulink Function : Subsystem  TreatAsAtomicUnit=on
  wires:
  Function-Call Generator/1 -> Function-Call Subsystem/Trigger

== system LLC_Controller/LLC Control/Fast_Sc_Ov_Protection ==
  function : TriggerPort  TriggerType=function-call  VariantControl=(inherit)

== system LLC_Controller/LLC Control/LLC_On_Off_Control ==
  function : TriggerPort  TriggerType=function-call  VariantControl=(inherit)
  Data Store Read1 : DataStoreRead  DataStoreName=LLC_Enable  IndexOptions=Index vector (dialog)  Indices=1  OutputSizes=1
  If : If  IfExpression=u1 == 1
  Subsystem_llc_off : Subsystem  TreatAsAtomicUnit=on
  Subsystem_llc_on : Subsystem  TreatAsAtomicUnit=on
  wires:
  If/2 -> Subsystem_llc_off/Action
  Data Store Read1/1 -> If/1
  If/1 -> Subsystem_llc_on/Action

== system LLC_Controller/LLC Control/Period_Update ==
  function : TriggerPort  TriggerType=function-call  VariantControl=(inherit)
  Function-Call Generator : simulink/Ports & Subsystems/Function-Call Generator  sample_time=-1  numberOfIterations=1  DisallowWideOutput=off
  Function-Call Split : FunctionCallSplit  NumOutputPorts=2
  Function-Call Subsystem : Subsystem  TreatAsAtomicUnit=on
  Function-Call Subsystem1 : Subsystem  TreatAsAtomicUnit=on
  wires:
  Function-Call Generator/1 -> Function-Call Split/1
  Function-Call Split/1 -> Function-Call Subsystem/Trigger
  Function-Call Split/2 -> Function-Call Subsystem1/Trigger

== system LLC_Controller/MCU_Config/CMPSS//ANALOG Initialize ==

== system LLC_Controller/MCU_Config/PWM Initialize ==

== system LLC_Controller/Schedule_task_100ms/SCI_A_Transmit_function1 ==
  SCI_A_Transmit_VADC_Suffix : TriggerPort  TriggerType=function-call  IsSimulinkFunction=on  FunctionName=SCI_A_Transmit_VADC_Suffix  FunctionVisibility=scoped  VariantControl=(inherit)
  SCI Transmit : c280xlib/SCI Transmit  sciModule=A  dataHead=''  dataTail=10  blockingMode=on  outputStatus=off
  VADC : Constant  Value=[86 65 68 67]  OutDataTypeStr=uint8
  wires:
  VADC/1 -> SCI Transmit/1

== system LLC_Controller/Schedule_task_100ms/SCI_A_Transmit_function15 ==
  SCI_A_Transmit_VBAT_Suffix : TriggerPort  TriggerType=function-call  IsSimulinkFunction=on  FunctionName=SCI_A_Transmit_VBAT_Suffix  FunctionVisibility=scoped  VariantControl=(inherit)
  SCI Transmit : c280xlib/SCI Transmit  sciModule=A  dataHead=''  dataTail=10  blockingMode=on  outputStatus=off
  VBAT : Constant  Value=[86 66 65 84]  OutDataTypeStr=uint8
  wires:
  VBAT/1 -> SCI Transmit/1

== system LLC_Controller/Schedule_task_100ms/SCI_A_Transmit_function17 ==
  SCI_A_Transmit_Current_Suffix : TriggerPort  TriggerType=function-call  IsSimulinkFunction=on  FunctionName=SCI_A_Transmit_Current_Suffix  FunctionVisibility=scoped  VariantControl=(inherit)
  SCI Transmit : c280xlib/SCI Transmit  sciModule=A  dataHead=''  dataTail=10  blockingMode=on  outputStatus=off
  mA_Iout : Constant  Value=[109 65 95 73 111 117 116]  OutDataTypeStr=uint8
  wires:
  mA_Iout/1 -> SCI Transmit/1

== system LLC_Controller/Schedule_task_100ms/SCI_A_Transmit_function19 ==
  SCI_A_Transmit_Duty_Suffix : TriggerPort  TriggerType=function-call  IsSimulinkFunction=on  FunctionName=SCI_A_Transmit_Duty_Suffix  FunctionVisibility=scoped  VariantControl=(inherit)
  Duty : Constant  Value=[68 117 116 121 95 68 66]  OutDataTypeStr=uint8
  SCI Transmit : c280xlib/SCI Transmit  sciModule=A  dataHead=''  dataTail=10  blockingMode=on  outputStatus=off
  wires:
  Duty/1 -> SCI Transmit/1

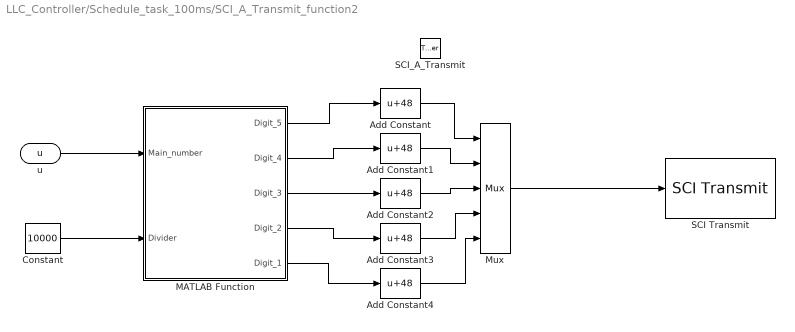
== system LLC_Controller/Schedule_task_100ms/SCI_A_Transmit_function2 ==
  SCI_A_Transmit : TriggerPort  TriggerType=function-call  IsSimulinkFunction=on  FunctionName=SCI_A_Transmit  FunctionVisibility=scoped  VariantControl=(inherit)
  Add Constant{,1..4} (5 alike) : Bias  Bias=48  SaturateOnIntegerOverflow=off
  Constant : Constant  Value=10000
  MATLAB Function : MATLAB Function  TreatAsAtomicUnit=on
  Mux : Mux  Inputs=5
  SCI Transmit : c280xlib/SCI Transmit  sciModule=A  dataHead=''  dataTail=''  blockingMode=on  outputStatus=off
  u : ArgIn  DisableCoverage=on  ArgumentName=u
  wires:
  u/1 -> MATLAB Function/1(Main_number)
  Constant/1 -> MATLAB Function/2(Divider)
  MATLAB Function/5(Digit_1) -> Add Constant4/1
  MATLAB Function/4(Digit_2) -> Add Constant3/1
  MATLAB Function/3(Digit_3) -> Add Constant2/1
  MATLAB Function/2(Digit_4) -> Add Constant1/1
  MATLAB Function/1(Digit_5) -> Add Constant/1
  Add Constant/1 -> Mux/1
  Add Constant1/1 -> Mux/2
  Add Constant2/1 -> Mux/3
  Add Constant3/1 -> Mux/4
  Add Constant4/1 -> Mux/5
  Mux/1 -> SCI Transmit/1

== system LLC_Controller/Schedule_task_100ms/SCI_A_Transmit_function21 ==
  SCI_A_Transmit_VBATRef_Suffix : TriggerPort  TriggerType=function-call  IsSimulinkFunction=on  FunctionName=SCI_A_Transmit_VBATRef_Suffix  FunctionVisibility=scoped  VariantControl=(inherit)
  SCI Transmit : c280xlib/SCI Transmit  sciModule=A  dataHead=''  dataTail=10  blockingMode=on  outputStatus=off
  VBATRef : Constant  Value=[86 66 65 84 82 101 102]  OutDataTypeStr=uint8
  wires:
  VBATRef/1 -> SCI Transmit/1

== system LLC_Controller/Schedule_task_100ms/SCI_A_Transmit_function22 ==
  SCI_A_Transmit_SS_Suffix : TriggerPort  TriggerType=function-call  IsSimulinkFunction=on  FunctionName=SCI_A_Transmit_SS_Suffix  FunctionVisibility=scoped  VariantControl=(inherit)
  SCI Transmit : c280xlib/SCI Transmit  sciModule=A  dataHead=''  dataTail=10  blockingMode=on  outputStatus=off
  SS : Constant  Value=[83 83]  OutDataTypeStr=uint8
  wires:
  SS/1 -> SCI Transmit/1

== system LLC_Controller/Schedule_task_100ms/SCI_A_Transmit_function23 ==
  SCI_A_Transmit_TBPHS_Suffix : TriggerPort  TriggerType=function-call  IsSimulinkFunction=on  FunctionName=SCI_A_Transmit_TBPHS_Suffix  FunctionVisibility=scoped  VariantControl=(inherit)
  SCI Transmit : c280xlib/SCI Transmit  sciModule=A  dataHead=''  dataTail=10  blockingMode=on  outputStatus=off
  TBPHS : Constant  Value=[84 66 80 72 83]  OutDataTypeStr=uint8
  wires:
  TBPHS/1 -> SCI Transmit/1

== system LLC_Controller/Schedule_task_100ms/SCI_A_Transmit_function24 ==
  SCI_A_Transmit_OCPFlag_Suffix : TriggerPort  TriggerType=function-call  IsSimulinkFunction=on  FunctionName=SCI_A_Transmit_OCPFlag_Suffix  FunctionVisibility=scoped  VariantControl=(inherit)
  OCPFlag : Constant  Value=[79 67 80 70 108 97 103]  OutDataTypeStr=uint8
  SCI Transmit : c280xlib/SCI Transmit  sciModule=A  dataHead=''  dataTail=10  blockingMode=on  outputStatus=off
  wires:
  OCPFlag/1 -> SCI Transmit/1

== system LLC_Controller/Schedule_task_100ms/SCI_A_Transmit_function25 ==
  SCI_A_Transmit_NewVRegPoint_Suffix : TriggerPort  TriggerType=function-call  IsSimulinkFunction=on  FunctionName=SCI_A_Transmit_NewVRegPoint_Suffix  FunctionVisibility=scoped  VariantControl=(inherit)
  NewVReg : Constant  Value=[78 101 119 86 82 101 103]  OutDataTypeStr=uint8
  SCI Transmit : c280xlib/SCI Transmit  sciModule=A  dataHead=''  dataTail=10  blockingMode=on  outputStatus=off
  wires:
  NewVReg/1 -> SCI Transmit/1

== system LLC_Controller/Schedule_task_100ms/SCI_A_Transmit_function3 ==
  SCI_A_Transmit_OVPFlag_Suffix : TriggerPort  TriggerType=function-call  IsSimulinkFunction=on  FunctionName=SCI_A_Transmit_OVPFlag_Suffix  FunctionVisibility=scoped  VariantControl=(inherit)
  OVPFlag : Constant  Value=[95 79 86 80 70 108 97 103]  OutDataTypeStr=uint8
  SCI Transmit : c280xlib/SCI Transmit  sciModule=A  dataHead=''  dataTail=10  blockingMode=on  outputStatus=off
  wires:
  OVPFlag/1 -> SCI Transmit/1

== system LLC_Controller/Schedule_task_100ms/SCI_A_Transmit_function4 ==
  SCI_A_Transmit_VAvg_Suffix : TriggerPort  TriggerType=function-call  IsSimulinkFunction=on  FunctionName=SCI_A_Transmit_VAvg_Suffix  FunctionVisibility=scoped  VariantControl=(inherit)
  SCI Transmit : c280xlib/SCI Transmit  sciModule=A  dataHead=''  dataTail=10  blockingMode=on  outputStatus=off
  VAvg : Constant  Value=[86 65 118 103]  OutDataTypeStr=uint8
  wires:
  VAvg/1 -> SCI Transmit/1

== system LLC_Controller/Schedule_task_100ms/SCI_A_Transmit_function5 ==
  SCI_A_Transmit_Freq_Suffix : TriggerPort  TriggerType=function-call  IsSimulinkFunction=on  FunctionName=SCI_A_Transmit_Freq_Suffix  FunctionVisibility=scoped  VariantControl=(inherit)
  KHz_FreqSend : Constant  Value=[75 72 122 95 70 114 101 113 83 101 110 100]  OutDataTypeStr=uint8
  SCI Transmit : c280xlib/SCI Transmit  sciModule=A  dataHead=''  dataTail=10  blockingMode=on  outputStatus=off
  wires:
  KHz_FreqSend/1 -> SCI Transmit/1

== system LLC_Controller/Schedule_task_100ms/SCI_A_Transmit_function6 ==
  SCI_A_Transmit_Vo_Suffix : TriggerPort  TriggerType=function-call  IsSimulinkFunction=on  FunctionName=SCI_A_Transmit_Vo_Suffix  FunctionVisibility=scoped  VariantControl=(inherit)
  SCI Transmit : c280xlib/SCI Transmit  sciModule=A  dataHead=''  dataTail=10  blockingMode=on  outputStatus=off
  Vo : Constant  Value=[86 111]  OutDataTypeStr=uint8
  wires:
  Vo/1 -> SCI Transmit/1

== system LLC_Controller/Schedule_task_100ms/SCI_A_Transmit_function7 ==
  SCI_A_Transmit_PFC_Suffix : TriggerPort  TriggerType=function-call  IsSimulinkFunction=on  FunctionName=SCI_A_Transmit_PFC_Suffix  FunctionVisibility=scoped  VariantControl=(inherit)
  PFC : Constant  Value=[80 70 67]  OutDataTypeStr=uint8
  SCI Transmit : c280xlib/SCI Transmit  sciModule=A  dataHead=''  dataTail=10  blockingMode=on  outputStatus=off
  wires:
  PFC/1 -> SCI Transmit/1

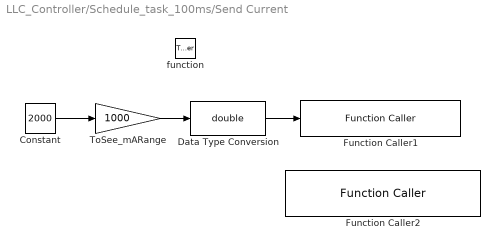
== system LLC_Controller/Schedule_task_100ms/Send Current ==
  function : TriggerPort  TriggerType=function-call  VariantControl=(inherit)
  Constant : Constant  Value=2000
  Data Type Conversion : DataTypeConversion  OutDataTypeStr=double  SaturateOnIntegerOverflow=off  RndMeth=Floor
  Function Caller1 : FunctionCaller  FunctionPrototype=SCI_A_Transmit(u)  InputArgumentSpecifications=<Enter example>  OutputArgumentSpecifications=<Enter example>
  Function Caller2 : FunctionCaller  FunctionPrototype=SCI_A_Transmit_Current_Suffix()  InputArgumentSpecifications=<Enter example>  OutputArgumentSpecifications=<Enter example>
  ToSee_mARange : Gain  Gain=1000
  wires:
  Data Type Conversion/1 -> Function Caller1/1
  Constant/1 -> ToSee_mARange/1
  ToSee_mARange/1 -> Data Type Conversion/1

== system LLC_Controller/Schedule_task_100ms/Send Duty ==
  function : TriggerPort  TriggerType=function-call  VariantControl=(inherit)
  Constant : Constant  Value=0
  Data Store Read1 : DataStoreRead  Commented=on  DataStoreName=Duty_Value  IndexOptions=Index vector (dialog)  Indices=1  OutputSizes=1
  Data Type Conversion : DataTypeConversion  OutDataTypeStr=double  SaturateOnIntegerOverflow=off  RndMeth=Floor
  Function Caller1 : FunctionCaller  FunctionPrototype=SCI_A_Transmit(u)  InputArgumentSpecifications=<Enter example>  OutputArgumentSpecifications=<Enter example>
  Function Caller2 : FunctionCaller  FunctionPrototype=SCI_A_Transmit_Duty_Suffix()  InputArgumentSpecifications=<Enter example>  OutputArgumentSpecifications=<Enter example>
  wires:
  Constant/1 -> Data Type Conversion/1
  Data Type Conversion/1 -> Function Caller1/1

== system LLC_Controller/Schedule_task_100ms/Send Freq ==
  function : TriggerPort  TriggerType=function-call  VariantControl=(inherit)
  Constant : Constant  Value=1000
  Data Type Conversion : DataTypeConversion  OutDataTypeStr=double  SaturateOnIntegerOverflow=off  RndMeth=Floor
  Function Caller1 : FunctionCaller  FunctionPrototype=SCI_A_Transmit(u)  InputArgumentSpecifications=<Enter example>  OutputArgumentSpecifications=<Enter example>
  Function Caller2 : FunctionCaller  FunctionPrototype=SCI_A_Transmit_Freq_Suffix()  InputArgumentSpecifications=<Enter example>  OutputArgumentSpecifications=<Enter example>
  wires:
  Constant/1 -> Data Type Conversion/1
  Data Type Conversion/1 -> Function Caller1/1

== system LLC_Controller/Schedule_task_100ms/Send NewVRegPoint ==
  function : TriggerPort  TriggerType=function-call  VariantControl=(inherit)
  Constant : Constant  Value=0
  Data Store Read1 : DataStoreRead  Commented=on  DataStoreName=VNewRegPoint  IndexOptions=Index vector (dialog)  Indices=1  OutputSizes=1
  Data Type Conversion : DataTypeConversion  OutDataTypeStr=double  SaturateOnIntegerOverflow=off  RndMeth=Floor
  Function Caller1 : FunctionCaller  FunctionPrototype=SCI_A_Transmit(u)  InputArgumentSpecifications=<Enter example>  OutputArgumentSpecifications=<Enter example>
  Function Caller2 : FunctionCaller  FunctionPrototype=SCI_A_Transmit_NewVRegPoint_Suffix()  InputArgumentSpecifications=<Enter example>  OutputArgumentSpecifications=<Enter example>
  wires:
  Constant/1 -> Data Type Conversion/1
  Data Type Conversion/1 -> Function Caller1/1

== system LLC_Controller/Schedule_task_100ms/Send OCPFlag ==
  function : TriggerPort  TriggerType=function-call  VariantControl=(inherit)
  Constant : Constant  Value=0
  Data Store Read1 : DataStoreRead  Commented=on  DataStoreName=OCP_Flag  IndexOptions=Index vector (dialog)  Indices=1  OutputSizes=1
  Data Type Conversion : DataTypeConversion  OutDataTypeStr=double  SaturateOnIntegerOverflow=off  RndMeth=Floor
  Function Caller1 : FunctionCaller  FunctionPrototype=SCI_A_Transmit(u)  InputArgumentSpecifications=<Enter example>  OutputArgumentSpecifications=<Enter example>
  Function Caller2 : FunctionCaller  FunctionPrototype=SCI_A_Transmit_OCPFlag_Suffix()  InputArgumentSpecifications=<Enter example>  OutputArgumentSpecifications=<Enter example>
  wires:
  Data Type Conversion/1 -> Function Caller1/1
  Constant/1 -> Data Type Conversion/1

== system LLC_Controller/Schedule_task_100ms/Send OVPFlag ==
  function : TriggerPort  TriggerType=function-call  VariantControl=(inherit)
  Constant : Constant  Value=0
  Data Store Read2 : DataStoreRead  Commented=on  DataStoreName=OVP_Flag  IndexOptions=Index vector (dialog)  Indices=1  OutputSizes=1
  Data Type Conversion : DataTypeConversion  OutDataTypeStr=double  SaturateOnIntegerOverflow=off  RndMeth=Floor
  Function Caller1 : FunctionCaller  FunctionPrototype=SCI_A_Transmit(u)  InputArgumentSpecifications=<Enter example>  OutputArgumentSpecifications=<Enter example>
  Function Caller2 : FunctionCaller  FunctionPrototype=SCI_A_Transmit_OVPFlag_Suffix()  InputArgumentSpecifications=<Enter example>  OutputArgumentSpecifications=<Enter example>
  wires:
  Constant/1 -> Data Type Conversion/1
  Data Type Conversion/1 -> Function Caller1/1

== system LLC_Controller/Schedule_task_100ms/Send PFC_OK ==
  function : TriggerPort  TriggerType=function-call  VariantControl=(inherit)
  Constant : Constant
  Data Store Read1 : DataStoreRead  Commented=on  DataStoreName=PFC_OK  IndexOptions=Index vector (dialog)  Indices=1  OutputSizes=1
  Data Type Conversion : DataTypeConversion  OutDataTypeStr=double  SaturateOnIntegerOverflow=off  RndMeth=Floor
  Function Caller1 : FunctionCaller  FunctionPrototype=SCI_A_Transmit(u)  InputArgumentSpecifications=<Enter example>  OutputArgumentSpecifications=<Enter example>
  Function Caller2 : FunctionCaller  FunctionPrototype=SCI_A_Transmit_PFC_Suffix()  InputArgumentSpecifications=<Enter example>  OutputArgumentSpecifications=<Enter example>
  wires:
  Data Type Conversion/1 -> Function Caller1/1
  Constant/1 -> Data Type Conversion/1

== system LLC_Controller/Schedule_task_100ms/Send SoftStart ==
  function : TriggerPort  TriggerType=function-call  VariantControl=(inherit)
  Constant : Constant  Value=0
  Data Store Read1 : DataStoreRead  Commented=on  DataStoreName=SoftStart_OK_Signal  IndexOptions=Index vector (dialog)  Indices=1  OutputSizes=1
  Data Type Conversion : DataTypeConversion  OutDataTypeStr=double  SaturateOnIntegerOverflow=off  RndMeth=Floor
  Function Caller1 : FunctionCaller  FunctionPrototype=SCI_A_Transmit(u)  InputArgumentSpecifications=<Enter example>  OutputArgumentSpecifications=<Enter example>
  Function Caller2 : FunctionCaller  FunctionPrototype=SCI_A_Transmit_SS_Suffix()  InputArgumentSpecifications=<Enter example>  OutputArgumentSpecifications=<Enter example>
  wires:
  Data Type Conversion/1 -> Function Caller1/1
  Constant/1 -> Data Type Conversion/1

== system LLC_Controller/Schedule_task_100ms/Send TBPHS (PhaseShift) ==
  function : TriggerPort  TriggerType=function-call  VariantControl=(inherit)
  Constant : Constant  Value=0
  Data Store Read1 : DataStoreRead  Commented=on  DataStoreName=TBPHS  IndexOptions=Index vector (dialog)  Indices=1  OutputSizes=1
  Data Type Conversion : DataTypeConversion  OutDataTypeStr=double  SaturateOnIntegerOverflow=off  RndMeth=Floor
  Function Caller1 : FunctionCaller  FunctionPrototype=SCI_A_Transmit(u)  InputArgumentSpecifications=<Enter example>  OutputArgumentSpecifications=<Enter example>
  Function Caller2 : FunctionCaller  FunctionPrototype=SCI_A_Transmit_TBPHS_Suffix()  InputArgumentSpecifications=<Enter example>  OutputArgumentSpecifications=<Enter example>
  wires:
  Constant/1 -> Data Type Conversion/1
  Data Type Conversion/1 -> Function Caller1/1

== system LLC_Controller/Schedule_task_100ms/Send VADC_Avg ==
  function : TriggerPort  TriggerType=function-call  VariantControl=(inherit)
  Constant : Constant
  Data Store Read1 : DataStoreRead  Commented=on  DataStoreName=VBAT_ADC_AvgValue  IndexOptions=Index vector (dialog)  Indices=1  OutputSizes=1
  Data Type Conversion : DataTypeConversion  Commented=on  OutDataTypeStr=double  SaturateOnIntegerOverflow=off  RndMeth=Floor
  Function Caller1 : FunctionCaller  FunctionPrototype=SCI_A_Transmit(u)  InputArgumentSpecifications=<Enter example>  OutputArgumentSpecifications=<Enter example>
  Function Caller2 : FunctionCaller  FunctionPrototype=SCI_A_Transmit_VAvg_Suffix()  InputArgumentSpecifications=<Enter example>  OutputArgumentSpecifications=<Enter example>
  wires:
  Constant/1 -> Function Caller1/1

== system LLC_Controller/Schedule_task_100ms/Send VBAT Value (Vout) ==
  function : TriggerPort  TriggerType=function-call  VariantControl=(inherit)
  Data Store Read : DataStoreRead  DataStoreName=Vbat_Adc  IndexOptions=Index vector (dialog)  Indices=1  OutputSizes=1
  Data Type Conversion : DataTypeConversion  OutDataTypeStr=double  SaturateOnIntegerOverflow=off  RndMeth=Floor
  Function Caller1 : FunctionCaller  FunctionPrototype=SCI_A_Transmit(u)  InputArgumentSpecifications=<Enter example>  OutputArgumentSpecifications=<Enter example>
  Function Caller2 : FunctionCaller  FunctionPrototype=SCI_A_Transmit_VBAT_Suffix()  InputArgumentSpecifications=<Enter example>  OutputArgumentSpecifications=<Enter example>
  wires:
  Data Type Conversion/1 -> Function Caller1/1
  Data Store Read/1 -> Data Type Conversion/1

== system LLC_Controller/Schedule_task_100ms/Send VBAT_Ref Value ==
  function : TriggerPort  TriggerType=function-call  VariantControl=(inherit)
  Data Store Read1 : DataStoreRead  DataStoreName=VBAT_Ref_Value  IndexOptions=Index vector (dialog)  Indices=1  OutputSizes=1
  Data Type Conversion : DataTypeConversion  OutDataTypeStr=double  SaturateOnIntegerOverflow=off  RndMeth=Floor
  Function Caller1 : FunctionCaller  FunctionPrototype=SCI_A_Transmit(u)  InputArgumentSpecifications=<Enter example>  OutputArgumentSpecifications=<Enter example>
  Function Caller2 : FunctionCaller  FunctionPrototype=SCI_A_Transmit_VBATRef_Suffix()  InputArgumentSpecifications=<Enter example>  OutputArgumentSpecifications=<Enter example>
  wires:
  Data Store Read1/1 -> Data Type Conversion/1
  Data Type Conversion/1 -> Function Caller1/1

== system LLC_Controller/Schedule_task_100ms/Send Vo Value ==
  function : TriggerPort  TriggerType=function-call  VariantControl=(inherit)
  Data Store Read1 : DataStoreRead  DataStoreName=Vo_Value  IndexOptions=Index vector (dialog)  Indices=1  OutputSizes=1
  Data Type Conversion : DataTypeConversion  OutDataTypeStr=double  SaturateOnIntegerOverflow=off  RndMeth=Floor
  Function Caller1 : FunctionCaller  FunctionPrototype=SCI_A_Transmit(u)  InputArgumentSpecifications=<Enter example>  OutputArgumentSpecifications=<Enter example>
  Function Caller2 : FunctionCaller  FunctionPrototype=SCI_A_Transmit_Vo_Suffix()  InputArgumentSpecifications=<Enter example>  OutputArgumentSpecifications=<Enter example>
  wires:
  Data Store Read1/1 -> Data Type Conversion/1
  Data Type Conversion/1 -> Function Caller1/1

== system LLC_Controller/Schedule_task_100ms/Send Voltage ADC Value ==
  function : TriggerPort  TriggerType=function-call  VariantControl=(inherit)
  Data Store Read1 : DataStoreRead  DataStoreName=VBAT_ADC_Value  IndexOptions=Index vector (dialog)  Indices=1  OutputSizes=1
  Data Type Conversion : DataTypeConversion  OutDataTypeStr=double  SaturateOnIntegerOverflow=off  RndMeth=Floor
  Function Caller1 : FunctionCaller  FunctionPrototype=SCI_A_Transmit(u)  InputArgumentSpecifications=<Enter example>  OutputArgumentSpecifications=<Enter example>
  Function Caller2 : FunctionCaller  FunctionPrototype=SCI_A_Transmit_VADC_Suffix()  InputArgumentSpecifications=<Enter example>  OutputArgumentSpecifications=<Enter example>
  wires:
  Data Store Read1/1 -> Data Type Conversion/1
  Data Type Conversion/1 -> Function Caller1/1

== system LLC_Controller/Schedule_task_1ms/Function-Call Subsystem1 ==
  function : TriggerPort  TriggerType=function-call  VariantControl=(inherit)
